simulink model "WaterRunner_open4"  (R2013a)
settings: Solver=ode23s  StartTime=0.0  StopTime=10  RelTol=1e-4
values from neighbouring files (symbols this model uses):
  dTorqueAmp = 1e-2    (= 0.01)    [SimParam_hopper.m]    (also in simParam.m = 0)
  dTorqueFreq = 0.5    [SimParam_hopper.m]    (also in simParam.m = 3.14159265359)
  dWaveAmp = 0    [simParam.m]
  dWaveFreq = (2*pi)/2    (= 3.14159265359)    [simParam.m]
  freq = findSSinput(y,b_water,k_water,A,Fratio,mass*g/4,w0)    [SimParam_hopper.m]    (also in findParams.m = freqs(k); simParam.m; sweepDFomega.m = FREQ(k))
  omega_0 = freq*ones(8,1)    [SimParam_hopper.m]    (also in findParams.m = freq*ones(4,1); simParam.m = freq*ones(4,1); sweepDFomega.m = freq*ones(4,1))
  tail_density = CF_density    (= 1790)    [simParam.m]
  tail_length = 0.1    [simParam.m]
  w1 = freq/(2*df)    [findParams.m]    (also in sweepDFomega.m)
  w2 = freq/(2*(1-df))    [findParams.m]    (also in sweepDFomega.m)
undefined symbols (not defined in the file or in its folder): X, Y, Z
undefined symbols (not defined in the file): cw_FL_HL, cw_FR_FL, cw_FR_HR, cw_HR_HL, FL_HL_lag, FR_FL_lag, FR_HR_lag, HR_HL_lag, phi0, tail_pad_radius, theta0, water_level, y0
libraries: nesl_utility x35, sm_lib x34, WaterRunner_lib_2 x11, simulink x2
(part 2 of 4)

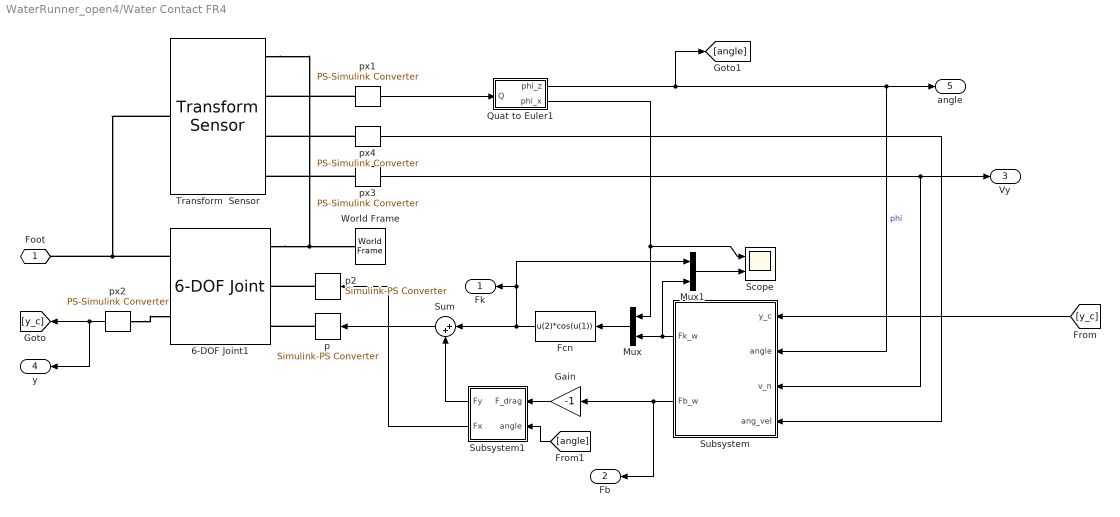
== system WaterRunner_open4/Water Contact FR4 ==
  6-DOF Joint1 : sm_lib/Joints/6-DOF Joint  SenseConstraintForceX=off  SenseConstraintForceY=off  SenseConstraintForceZ=off  SenseConstraintTorqueX=off  SenseConstraintTorqueY=off  SenseConstraintTorqueZ=off  ConstraintWrenchDir=FollowerOnBase  ConstraintWrenchFrame=BaseFrame  PxEquilibriumPosition=0  PxEquilibriumPositionUnits=m  PxSpringStiffness=0  PxSpringStiffnessUnits=N/m  PxDampingCoefficient=0  PxDampingCoefficientUnits=N/(m/s)  PxActuationMode=TorqueForceActuation  PxSensePosition=off  PxSenseVelocity=off  PxSenseAcceleration=off  PxSenseTorqueForce=off  PxPositionTargetValue=0  PxPositionTargetValueUnits=m  PxPositionTargetSpecify=off  PxPositionTargetPriority=High  PxVelocityTargetValue=0  PxVelocityTargetValueUnits=m/s  PxVelocityTargetSpecify=off  PxVelocityTargetPriority=High  PyEquilibriumPosition=0  PyEquilibriumPositionUnits=m  PySpringStiffness=0  PySpringStiffnessUnits=N/m  PyDampingCoefficient=0  PyDampingCoefficientUnits=N/(m/s)  PyActuationMode=TorqueForceActuation  PySensePosition=on  PySenseVelocity=off  PySenseAcceleration=off  PySenseTorqueForce=off  PyPositionTargetValue=0  PyPositionTargetValueUnits=m  PyPositionTargetSpecify=off  PyPositionTargetPriority=High  PyVelocityTargetValue=0  PyVelocityTargetValueUnits=m/s  PyVelocityTargetSpecify=off  PyVelocityTargetPriority=High  PzEquilibriumPosition=0  PzEquilibriumPositionUnits=m  PzSpringStiffness=0  PzSpringStiffnessUnits=N/m  PzDampingCoefficient=0  PzDampingCoefficientUnits=N/(m/s)  PzActuationMode=NoActuation  PzSensePosition=off  PzSenseVelocity=off  PzSenseAcceleration=off  PzSenseTorqueForce=off  PzPositionTargetValue=0  PzPositionTargetValueUnits=m  PzPositionTargetSpecify=off  PzPositionTargetPriority=High  PzVelocityTargetValue=0  PzVelocityTargetValueUnits=m/s  PzVelocityTargetSpecify=off  PzVelocityTargetPriority=High  SphDefPosRotationMethod=None  SphDefPosRotationAngleUnits=deg  SphDefPosRotationStandardAxis=+Z  SphDefPosRotationAngle=0  SphDefPosRotationArbitraryAxis=[0 0 1]  SphDefPosFollAlignAxisA=+X  SphDefPosBaseAlignAxisA=+Y  SphDefPosFollAlignAxisB=+Y  SphDefPosBaseAlignAxisB=+Z  SphEqPosRotationMethod=None  SphEqPosRotationAngleUnits=deg  SphEqPosRotationStandardAxis=+Z  SphEqPosRotationAngle=0  SphEqPosRotationArbitraryAxis=[0 0 1]  SphEqPosFollAlignAxisA=+X  SphEqPosBaseAlignAxisA=+Y  SphEqPosFollAlignAxisB=+Y  SphEqPosBaseAlignAxisB=+Z  SphSpringStiffness=0  SphSpringStiffnessUnits=N*m/deg  SphDampingCoefficient=0  SphDampingCoefficientUnits=N*m/(deg/s)  SphActuateTorqueX=off  SphActuateTorqueY=off  SphActuateTorqueZ=off  SphActuateTorque=off  SphActuationMode=NoActuation  SphActuationFrame=BaseFrame  SphSensePosition=off  SphSenseVelocityX=off  SphSenseVelocityY=off  SphSenseVelocityZ=off  SphSenseVelocity=off  SphSenseAccelerationX=off  SphSenseAccelerationY=off  SphSenseAccelerationZ=off  SphSenseAcceleration=off  SphSenseTorqueX=off  SphSenseTorqueY=off  SphSenseTorqueZ=off  SphSenseTorqueForce=off  SphSensingFrame=BaseFrame  SphPositionTargetRotationMethod=None  SphPositionTargetRotationAngleUnits=deg  SphPositionTargetRotationStandardAxis=+Z  SphPositionTargetRotationAngle=0  SphPositionTargetRotationArbitraryAxis=[0 0 1]  SphPositionTargetFollAlignAxisA=+X  SphPositionTargetBaseAlignAxisA=+Y  SphPositionTargetFollAlignAxisB=+Y  SphPositionTargetBaseAlignAxisB=+Z  SphPositionTargetSpecify=off  SphPositionTargetPriority=High  SphVelocityTargetValue=[0 0 0]  SphVelocityTargetValueUnits=deg/s  SphVelocityTargetSpecify=off  SphVelocityTargetPriority=High  SphVelocityTargetInFollowerFrame=on  BlockFunction=simmechanics.library.joints.sixdof_joint
  Fcn : Fcn  Expr=u(2)*cos(u(1))
  Gain : Gain  Gain=-1
  Mux : Mux  Inputs=2
  Mux1 : Mux  Inputs=2
  Quat to Euler1 : Subsystem
  Scope : Scope  NumInputPorts=2
      settings: YMin=-0.19~0  YMax=0.04~0.7  SaveName=ScopeData3
  Subsystem : Subsystem
  Subsystem1 : Subsystem
  Sum : Sum  Inputs=|++
  Transform  Sensor : sm_lib/Frames and  Transforms/Transform  Sensor  MeasurementFrame=NonRotatingBase  SenseAngle=off  SenseAxis=off  SenseAngle1=off  SenseAngle2=off  SenseAngle3=off  SenseQ=on  SenseR=off  SenseOmegaX=off  SenseOmegaY=off  SenseOmegaZ=on  SenseOmega1=off  SenseOmega2=off  SenseOmega3=off  SenseQDot=off  SenseRDot=off  SenseAlphaX=off  SenseAlphaY=off  SenseAlphaZ=off  SenseAlpha1=off  SenseAlpha2=off  SenseAlpha3=off  SenseQDDot=off  SenseRDDot=off  SenseX=off  SenseY=off  SenseZ=off  SenseRad=off  SenseAzim=off  SenseDist=off  SenseInc=off  SenseXDot=off  SenseYDot=on  SenseZDot=off  SenseRadDot=off  SenseAzimDot=off  SenseDistDot=off  SenseIncDot=off  SenseXDDot=off  SenseYDDot=off  SenseZDDot=off  SenseRadDDot=off  SenseAzimDDot=off  SenseDistDDot=off  SenseIncDDot=off  BlockFunction=simmechanics.library.frames_transforms.transform_sensor
  World Frame : sm_lib/Frames and  Transforms/World Frame  BlockFunction=simmechanics.library.frames_transforms.world_frame
  p : nesl_utility/Simulink-PS Converter  PhysicalDomain=network_engine_domain  SubClassName=ps_input  LeftPortType=input  RightPortType=output  PseudoPeriodic=off  Frequencies=[]  NoiseDistribution=none  NoiseParameters=[]  Unit=1  AffineConversion=off  InputFiltering=off  SimscapeFilterOrder=1  InputFilterTimeConstant=.001  UdotUserProvided=[]
  p2 : nesl_utility/Simulink-PS Converter  PhysicalDomain=network_engine_domain  SubClassName=ps_input  LeftPortType=input  RightPortType=output  PseudoPeriodic=off  Frequencies=[]  NoiseDistribution=none  NoiseParameters=[]  Unit=1  AffineConversion=off  InputFiltering=off  SimscapeFilterOrder=1  InputFilterTimeConstant=.001  UdotUserProvided=[]
  px{1..4} (4 alike) : nesl_utility/PS-Simulink Converter  PhysicalDomain=network_engine_domain  SubClassName=ps_output  LeftPortType=input  RightPortType=output  PseudoPeriodic=off  Frequencies=[]  Unit=1  AffineConversion=off
  Foot : PMIOPort  Port=1  Side=Left
  Fk : Outport
  Fb : Outport  Port=2
  Vy : Outport  Port=3
  y : Outport  Port=4
  angle : Outport  Port=5
  wires:
  Subsystem/2(Fb_w) -> Gain/1, Fb/1
  px3/1 -> Vy/1, Subsystem/3(v_n)
  Quat to Euler1/1(phi_z) -> [angle], Subsystem/2(angle), angle/1  "phi"
  px1/1 -> Quat to Euler1/1(Q)
  px4/1 -> Subsystem/4(ang_vel)
  px2/1 -> [y_c], y/1
  [angle] -> Subsystem1/2(angle)
  Sum/1 -> p/1
  Subsystem1/1(Fy) -> Sum/2
  Gain/1 -> Subsystem1/1(F_drag)
  Subsystem1/2(Fx) -> p2/1
  Subsystem/1(Fk_w) -> Mux1/2, Mux/2
  Mux/1 -> Fcn/1
  Fcn/1 -> Mux1/1, Fk/1, Sum/1
  Quat to Euler1/2(phi_x) -> Mux/1, Scope/1
  Mux1/1 -> Scope/2
  [y_c] -> Subsystem/1(y_c)
  connections:
  Transform  Sensor/RConn1 -- World Frame/RConn1 -- 6-DOF Joint1/LConn1
  Transform  Sensor/LConn1 -- Foot/RConn1 -- 6-DOF Joint1/RConn1
  px2/LConn1 -- 6-DOF Joint1/RConn2
  p/RConn1 -- 6-DOF Joint1/LConn3
  px1/LConn1 -- Transform  Sensor/RConn2
  p2/RConn1 -- 6-DOF Joint1/LConn2
  px3/LConn1 -- Transform  Sensor/RConn4
  px4/LConn1 -- Transform  Sensor/RConn3

== system WaterRunner_open4/observer ==
  Gain : Gain  Gain=-1
  Integrator : Integrator
  Integrator1 : Integrator
  Mux : Mux  Inputs=2
  Mux5 : Mux  Inputs=2
  PS-Simulink Converter : nesl_utility/PS-Simulink Converter  PhysicalDomain=network_engine_domain  SubClassName=ps_output  LeftPortType=input  RightPortType=output  PseudoPeriodic=off  Frequencies=[]  Unit=1  AffineConversion=off
  PS-Simulink Converter1 : nesl_utility/PS-Simulink Converter  PhysicalDomain=network_engine_domain  SubClassName=ps_output  LeftPortType=input  RightPortType=output  PseudoPeriodic=off  Frequencies=[]  Unit=1  AffineConversion=off
  PS-Simulink Converter2 : nesl_utility/PS-Simulink Converter  PhysicalDomain=network_engine_domain  SubClassName=ps_output  LeftPortType=input  RightPortType=output  PseudoPeriodic=off  Frequencies=[]  Unit=1  AffineConversion=off
  Transform  Sensor : sm_lib/Frames and  Transforms/Transform  Sensor  MeasurementFrame=World  SenseAngle=off  SenseAxis=off  SenseAngle1=off  SenseAngle2=off  SenseAngle3=off  SenseQ=off  SenseR=off  SenseOmegaX=on  SenseOmegaY=off  SenseOmegaZ=on  SenseOmega1=off  SenseOmega2=off  SenseOmega3=off  SenseQDot=off  SenseRDot=off  SenseAlphaX=off  SenseAlphaY=off  SenseAlphaZ=off  SenseAlpha1=off  SenseAlpha2=off  SenseAlpha3=off  SenseQDDot=off  SenseRDDot=off  SenseX=off  SenseY=on  SenseZ=off  SenseRad=off  SenseAzim=off  SenseDist=off  SenseInc=off  SenseXDot=off  SenseYDot=off  SenseZDot=off  SenseRadDot=off  SenseAzimDot=off  SenseDistDot=off  SenseIncDot=off  SenseXDDot=off  SenseYDDot=off  SenseZDDot=off  SenseRadDDot=off  SenseAzimDDot=off  SenseDistDDot=off  SenseIncDDot=off  BlockFunction=simmechanics.library.frames_transforms.transform_sensor
  averaging1 : Subsystem  mask{T_win=2*pi/freq, x_init=y0}
      mask prompts: T_win "window (s)"; x_init "Initial condition"
  averaging5 : Subsystem  mask{T_win=2*pi/freq, x_init=[theta0 phi0]}
      mask prompts: T_win "window (s)"; x_init "Initial condition"
  Base : PMIOPort  Port=1  Side=Left
  Follower : PMIOPort  Port=2  Side=Left
  output : Outport
  wires:
  Mux5/1 -> output/1
  Mux/1 -> averaging5/1(in)
  PS-Simulink Converter/1 -> Integrator/1
  Integrator1/1 -> Mux/2
  Integrator/1 -> Gain/1
  PS-Simulink Converter1/1 -> Integrator1/1
  PS-Simulink Converter2/1 -> averaging1/1(in)
  averaging1/1(out) -> Mux5/1
  averaging5/1(out) -> Mux5/2
  Gain/1 -> Mux/1
  connections:
  Transform  Sensor/LConn1 -- Base/RConn1
  PS-Simulink Converter/LConn1 -- Transform  Sensor/RConn2
  Follower/RConn1 -- Transform  Sensor/RConn1
  PS-Simulink Converter1/LConn1 -- Transform  Sensor/RConn3
  PS-Simulink Converter2/LConn1 -- Transform  Sensor/RConn4

== system WaterRunner_open4/CPG_Network/FL_HL lag ==
  In1 : Inport
  In2 : Inport  Port=2
  Constant : Constant  Value=d_phase
  Gain : Gain  Gain=-1
  Sum : Sum  Inputs=--+
  sin : Fcn  Expr=coupling_weight*sin(u(1))
  Out1 : Outport
  Out2 : Outport  Port=2
  wires:
  Sum/1 -> sin/1
  sin/1 -> Gain/1, Out1/1
  Constant/1 -> Sum/2
  In1/1 -> Sum/1
  In2/1 -> Sum/3
  Gain/1 -> Out2/1

== system WaterRunner_open4/CPG_Network/FR_FL lag ==
  In1 : Inport
  In2 : Inport  Port=2
  Constant : Constant  Value=d_phase
  Gain : Gain  Gain=-1
  Sum : Sum  Inputs=--+
  sin : Fcn  Expr=coupling_weight*sin(u(1))
  Out1 : Outport
  Out2 : Outport  Port=2
  wires:
  Sum/1 -> sin/1
  sin/1 -> Gain/1, Out1/1
  Constant/1 -> Sum/2
  In1/1 -> Sum/1
  In2/1 -> Sum/3
  Gain/1 -> Out2/1

== system WaterRunner_open4/CPG_Network/FR_HR lag ==
  In1 : Inport
  In2 : Inport  Port=2
  Constant : Constant  Value=d_phase
  Gain : Gain  Gain=-1
  Sum : Sum  Inputs=--+
  sin : Fcn  Expr=coupling_weight*sin(u(1))
  Out1 : Outport
  Out2 : Outport  Port=2
  wires:
  Gain/1 -> Out2/1
  In2/1 -> Sum/3
  In1/1 -> Sum/1
  Constant/1 -> Sum/2
  sin/1 -> Out1/1, Gain/1
  Sum/1 -> sin/1

== system WaterRunner_open4/CPG_Network/Front_Left ==
  force : Inport
  Constant3 : Constant  Value=freq
  Integrator3 : Integrator  InitialCondition=init_phi + 0.001*rand
  Mod 2pi : Fcn  Expr=atan2(sin(u(1)-pi),cos(u(1)-pi))+pi
  Sum2 : Sum  Inputs=|++
  vel : Outport
  phase : Outport  Port=2
  wires:
  force/1 -> Sum2/2
  Sum2/1 -> vel/1, Integrator3/1
  Constant3/1 -> Sum2/1
  Integrator3/1 -> Mod 2pi/1
  Mod 2pi/1 -> phase/1

== system WaterRunner_open4/CPG_Network/Front_Right ==
  force : Inport
  Constant3 : Constant  Value=freq
  Integrator3 : Integrator  InitialCondition=init_phi + 0.001*rand
  Mod 2pi : Fcn  Expr=atan2(sin(u(1)-pi),cos(u(1)-pi))+pi
  Sum2 : Sum  Inputs=|++
  vel : Outport
  phase : Outport  Port=2
  wires:
  Mod 2pi/1 -> phase/1
  Integrator3/1 -> Mod 2pi/1
  Constant3/1 -> Sum2/1
  Sum2/1 -> Integrator3/1, vel/1
  force/1 -> Sum2/2

== system WaterRunner_open4/CPG_Network/HR_HL lag ==
  In1 : Inport
  In2 : Inport  Port=2
  Constant : Constant  Value=d_phase
  Gain : Gain  Gain=-1
  Sum : Sum  Inputs=--+
  sin : Fcn  Expr=coupling_weight*sin(u(1))
  Out1 : Outport
  Out2 : Outport  Port=2
  wires:
  Gain/1 -> Out2/1
  In2/1 -> Sum/3
  In1/1 -> Sum/1
  Constant/1 -> Sum/2
  sin/1 -> Out1/1, Gain/1
  Sum/1 -> sin/1

== system WaterRunner_open4/CPG_Network/Hind_Left ==
  force : Inport
  Constant3 : Constant  Value=freq
  Integrator3 : Integrator  InitialCondition=init_phi + 0.001*rand
  Mod 2pi : Fcn  Expr=atan2(sin(u(1)-pi),cos(u(1)-pi))+pi
  Sum2 : Sum  Inputs=|++
  vel : Outport
  phase : Outport  Port=2
  wires:
  force/1 -> Sum2/2
  Sum2/1 -> vel/1, Integrator3/1
  Constant3/1 -> Sum2/1
  Integrator3/1 -> Mod 2pi/1
  Mod 2pi/1 -> phase/1

== system WaterRunner_open4/CPG_Network/Hind_Right ==
  force : Inport
  Constant3 : Constant  Value=freq
  Integrator3 : Integrator  InitialCondition=init_phi + 0.001*rand
  Mod 2pi : Fcn  Expr=atan2(sin(u(1)-pi),cos(u(1)-pi))+pi
  Sum2 : Sum  Inputs=|++
  vel : Outport
  phase : Outport  Port=2
  wires:
  force/1 -> Sum2/2
  Sum2/1 -> vel/1, Integrator3/1
  Constant3/1 -> Sum2/1
  Integrator3/1 -> Mod 2pi/1
  Mod 2pi/1 -> phase/1

== system WaterRunner_open4/CPG_Network/split FL ==
  w_pos : Inport
  phase : Inport  Port=2
  w_neg : Inport  Port=3
  Product : Product  RndMeth=Zero
  Product1 : Product  RndMeth=Zero
  Sum2 : Sum  Inputs=|++
  enable : Subsystem
  Force : Outport
  wires:
  Product/1 -> Sum2/1
  w_pos/1 -> Product/1
  w_neg/1 -> Product1/1
  Product1/1 -> Sum2/2
  enable/1(pos) -> Product/2
  enable/2(neg) -> Product1/2
  Sum2/1 -> Force/1
  phase/1 -> enable/1(in)

== system WaterRunner_open4/CPG_Network/split FL1 ==
  w_pos : Inport
  phase : Inport  Port=2
  w_neg : Inport  Port=3
  Product : Product  RndMeth=Zero
  Product1 : Product  RndMeth=Zero
  Sum2 : Sum  Inputs=|++
  enable : Subsystem
  Force : Outport
  wires:
  Product/1 -> Sum2/1
  w_pos/1 -> Product/1
  w_neg/1 -> Product1/1
  Product1/1 -> Sum2/2
  enable/1(pos) -> Product/2
  enable/2(neg) -> Product1/2
  Sum2/1 -> Force/1
  phase/1 -> enable/1(in)

== system WaterRunner_open4/CPG_Network/split FL2 ==
  w_pos : Inport
  phase : Inport  Port=2
  w_neg : Inport  Port=3
  Product : Product  RndMeth=Zero
  Product1 : Product  RndMeth=Zero
  Sum2 : Sum  Inputs=|++
  enable : Subsystem
  Force : Outport
  wires:
  phase/1 -> enable/1(in)
  Sum2/1 -> Force/1
  enable/2(neg) -> Product1/2
  enable/1(pos) -> Product/2
  Product1/1 -> Sum2/2
  w_neg/1 -> Product1/1
  w_pos/1 -> Product/1
  Product/1 -> Sum2/1

== system WaterRunner_open4/CPG_Network/split FL3 ==
  w_pos : Inport
  phase : Inport  Port=2
  w_neg : Inport  Port=3
  Product : Product  RndMeth=Zero
  Product1 : Product  RndMeth=Zero
  Sum2 : Sum  Inputs=|++
  enable : Subsystem
  Force : Outport
  wires:
  Product/1 -> Sum2/1
  w_pos/1 -> Product/1
  w_neg/1 -> Product1/1
  Product1/1 -> Sum2/2
  enable/1(pos) -> Product/2
  enable/2(neg) -> Product1/2
  Sum2/1 -> Force/1
  phase/1 -> enable/1(in)

== system WaterRunner_open4/Tail/Water Contact HR1 ==
  6-DOF Joint2 : sm_lib/Joints/6-DOF Joint  SenseConstraintForceX=off  SenseConstraintForceY=off  SenseConstraintForceZ=off  SenseConstraintTorqueX=off  SenseConstraintTorqueY=off  SenseConstraintTorqueZ=off  ConstraintWrenchDir=FollowerOnBase  ConstraintWrenchFrame=BaseFrame  PxEquilibriumPosition=0  PxEquilibriumPositionUnits=m  PxSpringStiffness=0  PxSpringStiffnessUnits=N/m  PxDampingCoefficient=0  PxDampingCoefficientUnits=N/(m/s)  PxActuationMode=TorqueForceActuation  PxSensePosition=off  PxSenseVelocity=off  PxSenseAcceleration=off  PxSenseTorqueForce=off  PxPositionTargetValue=0  PxPositionTargetValueUnits=m  PxPositionTargetSpecify=off  PxPositionTargetPriority=High  PxVelocityTargetValue=0  PxVelocityTargetValueUnits=m/s  PxVelocityTargetSpecify=off  PxVelocityTargetPriority=High  PyEquilibriumPosition=0  PyEquilibriumPositionUnits=m  PySpringStiffness=0  PySpringStiffnessUnits=N/m  PyDampingCoefficient=0  PyDampingCoefficientUnits=N/(m/s)  PyActuationMode=TorqueForceActuation  PySensePosition=on  PySenseVelocity=off  PySenseAcceleration=off  PySenseTorqueForce=off  PyPositionTargetValue=0  PyPositionTargetValueUnits=m  PyPositionTargetSpecify=off  PyPositionTargetPriority=High  PyVelocityTargetValue=0  PyVelocityTargetValueUnits=m/s  PyVelocityTargetSpecify=off  PyVelocityTargetPriority=High  PzEquilibriumPosition=0  PzEquilibriumPositionUnits=m  PzSpringStiffness=0  PzSpringStiffnessUnits=N/m  PzDampingCoefficient=0  PzDampingCoefficientUnits=N/(m/s)  PzActuationMode=NoActuation  PzSensePosition=off  PzSenseVelocity=off  PzSenseAcceleration=off  PzSenseTorqueForce=off  PzPositionTargetValue=0  PzPositionTargetValueUnits=m  PzPositionTargetSpecify=off  PzPositionTargetPriority=High  PzVelocityTargetValue=0  PzVelocityTargetValueUnits=m/s  PzVelocityTargetSpecify=off  PzVelocityTargetPriority=High  SphDefPosRotationMethod=None  SphDefPosRotationAngleUnits=deg  SphDefPosRotationStandardAxis=+Z  SphDefPosRotationAngle=0  SphDefPosRotationArbitraryAxis=[0 0 1]  SphDefPosFollAlignAxisA=+X  SphDefPosBaseAlignAxisA=+Y  SphDefPosFollAlignAxisB=+Y  SphDefPosBaseAlignAxisB=+Z  SphEqPosRotationMethod=None  SphEqPosRotationAngleUnits=deg  SphEqPosRotationStandardAxis=+Z  SphEqPosRotationAngle=0  SphEqPosRotationArbitraryAxis=[0 0 1]  SphEqPosFollAlignAxisA=+X  SphEqPosBaseAlignAxisA=+Y  SphEqPosFollAlignAxisB=+Y  SphEqPosBaseAlignAxisB=+Z  SphSpringStiffness=0  SphSpringStiffnessUnits=N*m/deg  SphDampingCoefficient=0  SphDampingCoefficientUnits=N*m/(deg/s)  SphActuateTorqueX=off  SphActuateTorqueY=off  SphActuateTorqueZ=off  SphActuateTorque=off  SphActuationMode=NoActuation  SphActuationFrame=BaseFrame  SphSensePosition=off  SphSenseVelocityX=off  SphSenseVelocityY=off  SphSenseVelocityZ=off  SphSenseVelocity=off  SphSenseAccelerationX=off  SphSenseAccelerationY=off  SphSenseAccelerationZ=off  SphSenseAcceleration=off  SphSenseTorqueX=off  SphSenseTorqueY=off  SphSenseTorqueZ=off  SphSenseTorqueForce=off  SphSensingFrame=BaseFrame  SphPositionTargetRotationMethod=None  SphPositionTargetRotationAngleUnits=deg  SphPositionTargetRotationStandardAxis=+Z  SphPositionTargetRotationAngle=0  SphPositionTargetRotationArbitraryAxis=[0 0 1]  SphPositionTargetFollAlignAxisA=+X  SphPositionTargetBaseAlignAxisA=+Y  SphPositionTargetFollAlignAxisB=+Y  SphPositionTargetBaseAlignAxisB=+Z  SphPositionTargetSpecify=off  SphPositionTargetPriority=High  SphVelocityTargetValue=[0 0 0]  SphVelocityTargetValueUnits=deg/s  SphVelocityTargetSpecify=off  SphVelocityTargetPriority=High  SphVelocityTargetInFollowerFrame=on  BlockFunction=simmechanics.library.joints.sixdof_joint
  Gain : Gain  Gain=-1
  Gain1 : Gain  Gain=-1
  Quat to Euler1 : WaterRunner_lib_2/Water Contact FR/Quat to Euler1
  Subsystem1 : WaterRunner_lib_2/Water Contact FR/Subsystem1
  Transform  Sensor : sm_lib/Frames and  Transforms/Transform  Sensor  MeasurementFrame=NonRotatingBase  SenseAngle=off  SenseAxis=off  SenseAngle1=off  SenseAngle2=off  SenseAngle3=off  SenseQ=on  SenseR=off  SenseOmegaX=off  SenseOmegaY=off  SenseOmegaZ=on  SenseOmega1=off  SenseOmega2=off  SenseOmega3=off  SenseQDot=off  SenseRDot=off  SenseAlphaX=off  SenseAlphaY=off  SenseAlphaZ=off  SenseAlpha1=off  SenseAlpha2=off  SenseAlpha3=off  SenseQDDot=off  SenseRDDot=off  SenseX=off  SenseY=off  SenseZ=off  SenseRad=off  SenseAzim=off  SenseDist=off  SenseInc=off  SenseXDot=off  SenseYDot=on  SenseZDot=off  SenseRadDot=off  SenseAzimDot=off  SenseDistDot=off  SenseIncDot=off  SenseXDDot=off  SenseYDDot=off  SenseZDDot=off  SenseRadDDot=off  SenseAzimDDot=off  SenseDistDDot=off  SenseIncDDot=off  BlockFunction=simmechanics.library.frames_transforms.transform_sensor
  World Frame1 : sm_lib/Frames and  Transforms/World Frame  BlockFunction=simmechanics.library.frames_transforms.world_frame
  p : nesl_utility/Simulink-PS Converter  PhysicalDomain=network_engine_domain  SubClassName=ps_input  LeftPortType=input  RightPortType=output  PseudoPeriodic=off  Frequencies=[]  NoiseDistribution=none  NoiseParameters=[]  Unit=1  AffineConversion=off  InputFiltering=off  SimscapeFilterOrder=1  InputFilterTimeConstant=.001  UdotUserProvided=[]
  p2 : nesl_utility/Simulink-PS Converter  PhysicalDomain=network_engine_domain  SubClassName=ps_input  LeftPortType=input  RightPortType=output  PseudoPeriodic=off  Frequencies=[]  NoiseDistribution=none  NoiseParameters=[]  Unit=1  AffineConversion=off  InputFiltering=off  SimscapeFilterOrder=1  InputFilterTimeConstant=.001  UdotUserProvided=[]
  px{1..4} (4 alike) : nesl_utility/PS-Simulink Converter  PhysicalDomain=network_engine_domain  SubClassName=ps_output  LeftPortType=input  RightPortType=output  PseudoPeriodic=off  Frequencies=[]  Unit=1  AffineConversion=off
  water_model : Subsystem  mask{Cd=0.703, density=1000, y_w=water_level, R=tail_pad_radius, g=-9.81}
      mask prompts: Cd "Drag Coefficient"; y_w "Water level"; R "Foot Radius"; g "Gravity constant (use negative)"
  Foot : PMIOPort  Port=1  Side=Left
  Fb : Outport
  wires:
  water_model/1(Fb_w) -> Fb/1, Gain/1
  px3/1 -> water_model/3(v_n)
  Quat to Euler1/1 -> [angle], water_model/2(angle)  "phi"
  px1/1 -> Quat to Euler1/1
  px4/1 -> water_model/4(ang_vel)
  px2/1 -> [y_c]
  [y_c] -> water_model/1(y_c)
  [angle] -> Subsystem1/2
  Subsystem1/2 -> Gain1/1
  Subsystem1/1 -> p/1
  Gain/1 -> Subsystem1/1
  Gain1/1 -> p2/1
  connections:
  World Frame1/RConn1 -- Transform  Sensor/RConn1 -- 6-DOF Joint2/LConn1
  Transform  Sensor/LConn1 -- Foot/RConn1 -- 6-DOF Joint2/RConn1
  Transform  Sensor/RConn4 -- px3/LConn1
  px4/LConn1 -- Transform  Sensor/RConn3
  p2/RConn1 -- 6-DOF Joint2/LConn2
  p/RConn1 -- 6-DOF Joint2/LConn3
  px2/LConn1 -- 6-DOF Joint2/RConn2
  px1/LConn1 -- Transform  Sensor/RConn2

== system WaterRunner_open4/Water Contact FR1/Quat to Euler1 ==
  Q : Inport
  f1 : Fcn  Expr=atan2( 2*(u(1)*u(2) + u(3)*u(4)) , 1-2*(u(2)^2+u(3)^2) )
  f3 : Fcn  Expr=atan2( 2*(u(1)*u(4) + u(2)*u(3)) , 1-2*(u(3)^2+u(4)^2) )
  phi_z : Outport
  phi_x : Outport  Port=2
  wires:
  Q/1 -> f1/1, f3/1
  f3/1 -> phi_z/1
  f1/1 -> phi_x/1

== system WaterRunner_open4/Water Contact FR1/Subsystem ==
  y_c : Inport
  angle : Inport  Port=2
  v_n : Inport  Port=3
  ang_vel : Inport  Port=4
  Switch : Switch
  Switch1 : Switch
  water_model : Subsystem  mask{Cd=0.703, density=1000, y_w=water_level, R=0.02, g=-9.81}
      mask prompts: Cd "Drag Coefficient"; y_w "Water level"; R "Foot Radius"; g "Gravity constant (use negative)"
  water_model1 : Subsystem  mask{Cd=0.703, density=1000, y_w=water_level, R=0.005, g=-9.81}
      mask prompts: Cd "Drag Coefficient"; y_w "Water level"; R "Foot Radius"; g "Gravity constant (use negative)"
  Fk_w : Outport
  Fb_w : Outport  Port=2
  wires:
  angle/1 -> water_model1/2(angle), water_model/2(angle)
  ang_vel/1 -> water_model1/4(ang_vel), water_model/4(ang_vel)
  y_c/1 -> water_model1/1(y_c), water_model/1(y_c)
  v_n/1 -> water_model1/3(v_n), Switch/2, Switch1/2, water_model/3(v_n)
  water_model/1(Fk_w) -> Switch/1
  water_model/2(Fb_w) -> Switch1/1
  Switch/1 -> Fk_w/1
  water_model1/1(Fk_w) -> Switch/3
  water_model1/2(Fb_w) -> Switch1/3
  Switch1/1 -> Fb_w/1

== system WaterRunner_open4/Water Contact FR1/Subsystem1 ==
  F_drag : Inport
  angle : Inport  Port=2
  Mux : Mux  Inputs=2
  fcosq : Fcn  Expr=u(1)*cos(u(2))
  fsinq : Fcn  Expr=u(1)*sin(u(2))
  Fy : Outport
  Fx : Outport  Port=2
  wires:
  angle/1 -> Mux/2
  fcosq/1 -> Fy/1
  F_drag/1 -> Mux/1
  Mux/1 -> fcosq/1, fsinq/1
  fsinq/1 -> Fx/1

== system WaterRunner_open4/Water Contact FR2/Quat to Euler1 ==
  Q : Inport
  f1 : Fcn  Expr=atan2( 2*(u(1)*u(2) + u(3)*u(4)) , 1-2*(u(2)^2+u(3)^2) )
  f3 : Fcn  Expr=atan2( 2*(u(1)*u(4) + u(2)*u(3)) , 1-2*(u(3)^2+u(4)^2) )
  phi_z : Outport
  phi_x : Outport  Port=2
  wires:
  Q/1 -> f1/1, f3/1
  f3/1 -> phi_z/1
  f1/1 -> phi_x/1

== system WaterRunner_open4/Water Contact FR2/Subsystem ==
  y_c : Inport
  angle : Inport  Port=2
  v_n : Inport  Port=3
  ang_vel : Inport  Port=4
  Switch : Switch
  Switch1 : Switch
  water_model : Subsystem  mask{Cd=0.703, density=1000, y_w=water_level, R=0.02, g=-9.81}
      mask prompts: Cd "Drag Coefficient"; y_w "Water level"; R "Foot Radius"; g "Gravity constant (use negative)"
  water_model1 : Subsystem  mask{Cd=0.703, density=1000, y_w=water_level, R=0.005, g=-9.81}
      mask prompts: Cd "Drag Coefficient"; y_w "Water level"; R "Foot Radius"; g "Gravity constant (use negative)"
  Fk_w : Outport
  Fb_w : Outport  Port=2
  wires:
  angle/1 -> water_model1/2(angle), water_model/2(angle)
  ang_vel/1 -> water_model1/4(ang_vel), water_model/4(ang_vel)
  y_c/1 -> water_model1/1(y_c), water_model/1(y_c)
  v_n/1 -> water_model1/3(v_n), Switch/2, Switch1/2, water_model/3(v_n)
  water_model/1(Fk_w) -> Switch/1
  water_model/2(Fb_w) -> Switch1/1
  Switch/1 -> Fk_w/1
  water_model1/1(Fk_w) -> Switch/3
  water_model1/2(Fb_w) -> Switch1/3
  Switch1/1 -> Fb_w/1

== system WaterRunner_open4/Water Contact FR2/Subsystem1 ==
  F_drag : Inport
  angle : Inport  Port=2
  Mux : Mux  Inputs=2
  fcosq : Fcn  Expr=u(1)*cos(u(2))
  fsinq : Fcn  Expr=u(1)*sin(u(2))
  Fy : Outport
  Fx : Outport  Port=2
  wires:
  angle/1 -> Mux/2
  fcosq/1 -> Fy/1
  F_drag/1 -> Mux/1
  Mux/1 -> fcosq/1, fsinq/1
  fsinq/1 -> Fx/1

== system WaterRunner_open4/Water Contact FR3/Quat to Euler1 ==
  Q : Inport
  f1 : Fcn  Expr=atan2( 2*(u(1)*u(2) + u(3)*u(4)) , 1-2*(u(2)^2+u(3)^2) )
  f3 : Fcn  Expr=atan2( 2*(u(1)*u(4) + u(2)*u(3)) , 1-2*(u(3)^2+u(4)^2) )
  phi_z : Outport
  phi_x : Outport  Port=2
  wires:
  Q/1 -> f1/1, f3/1
  f3/1 -> phi_z/1
  f1/1 -> phi_x/1

== system WaterRunner_open4/Water Contact FR3/Subsystem ==
  y_c : Inport
  angle : Inport  Port=2
  v_n : Inport  Port=3
  ang_vel : Inport  Port=4
  Switch : Switch
  Switch1 : Switch
  water_model : Subsystem  mask{Cd=0.703, density=1000, y_w=water_level, R=0.02, g=-9.81}
      mask prompts: Cd "Drag Coefficient"; y_w "Water level"; R "Foot Radius"; g "Gravity constant (use negative)"
  water_model1 : Subsystem  mask{Cd=0.703, density=1000, y_w=water_level, R=0.005, g=-9.81}
      mask prompts: Cd "Drag Coefficient"; y_w "Water level"; R "Foot Radius"; g "Gravity constant (use negative)"
  Fk_w : Outport
  Fb_w : Outport  Port=2
  wires:
  angle/1 -> water_model1/2(angle), water_model/2(angle)
  ang_vel/1 -> water_model1/4(ang_vel), water_model/4(ang_vel)
  y_c/1 -> water_model1/1(y_c), water_model/1(y_c)
  v_n/1 -> water_model1/3(v_n), Switch/2, Switch1/2, water_model/3(v_n)
  water_model/1(Fk_w) -> Switch/1
  water_model/2(Fb_w) -> Switch1/1
  Switch/1 -> Fk_w/1
  water_model1/1(Fk_w) -> Switch/3
  water_model1/2(Fb_w) -> Switch1/3
  Switch1/1 -> Fb_w/1

== system WaterRunner_open4/Water Contact FR3/Subsystem1 ==
  F_drag : Inport
  angle : Inport  Port=2
  Mux : Mux  Inputs=2
  fcosq : Fcn  Expr=u(1)*cos(u(2))
  fsinq : Fcn  Expr=u(1)*sin(u(2))
  Fy : Outport
  Fx : Outport  Port=2
  wires:
  angle/1 -> Mux/2
  fcosq/1 -> Fy/1
  F_drag/1 -> Mux/1
  Mux/1 -> fcosq/1, fsinq/1
  fsinq/1 -> Fx/1

== system WaterRunner_open4/Water Contact FR4/Quat to Euler1 ==
  Q : Inport
  f1 : Fcn  Expr=atan2( 2*(u(1)*u(2) + u(3)*u(4)) , 1-2*(u(2)^2+u(3)^2) )
  f3 : Fcn  Expr=atan2( 2*(u(1)*u(4) + u(2)*u(3)) , 1-2*(u(3)^2+u(4)^2) )
  phi_z : Outport
  phi_x : Outport  Port=2
  wires:
  Q/1 -> f1/1, f3/1
  f3/1 -> phi_z/1
  f1/1 -> phi_x/1

== system WaterRunner_open4/Water Contact FR4/Subsystem ==
  y_c : Inport
  angle : Inport  Port=2
  v_n : Inport  Port=3
  ang_vel : Inport  Port=4
  Switch : Switch
  Switch1 : Switch
  water_model : Subsystem  mask{Cd=0.703, density=1000, y_w=water_level, R=0.02, g=-9.81}
      mask prompts: Cd "Drag Coefficient"; y_w "Water level"; R "Foot Radius"; g "Gravity constant (use negative)"
  water_model1 : Subsystem  mask{Cd=0.703, density=1000, y_w=water_level, R=0.005, g=-9.81}
      mask prompts: Cd "Drag Coefficient"; y_w "Water level"; R "Foot Radius"; g "Gravity constant (use negative)"
  Fk_w : Outport
  Fb_w : Outport  Port=2
  wires:
  angle/1 -> water_model1/2(angle), water_model/2(angle)
  ang_vel/1 -> water_model1/4(ang_vel), water_model/4(ang_vel)
  y_c/1 -> water_model1/1(y_c), water_model/1(y_c)
  v_n/1 -> water_model1/3(v_n), Switch/2, Switch1/2, water_model/3(v_n)
  water_model/1(Fk_w) -> Switch/1
  water_model/2(Fb_w) -> Switch1/1
  Switch/1 -> Fk_w/1
  water_model1/1(Fk_w) -> Switch/3
  water_model1/2(Fb_w) -> Switch1/3
  Switch1/1 -> Fb_w/1

== system WaterRunner_open4/Water Contact FR4/Subsystem1 ==
  F_drag : Inport
  angle : Inport  Port=2
  Mux : Mux  Inputs=2
  fcosq : Fcn  Expr=u(1)*cos(u(2))
  fsinq : Fcn  Expr=u(1)*sin(u(2))
  Fy : Outport
  Fx : Outport  Port=2
  wires:
  angle/1 -> Mux/2
  fcosq/1 -> Fy/1
  F_drag/1 -> Mux/1
  Mux/1 -> fcosq/1, fsinq/1
  fsinq/1 -> Fx/1

== system WaterRunner_open4/observer/averaging1 ==
  in : Inport
  Constant1 : Constant  Value=x_init
  Gain : Gain  Gain=1/T_win
  Integrator1 : Integrator
  Sum : Sum  Inputs=+-|
  Sum1 : Sum  Inputs=-+|
  Sum3 : Sum  Inputs=++|
  Transport Delay : TransportDelay  DelayTime=T_win
  out : Outport
  wires:
  in/1 -> Sum1/2
  Gain/1 -> Sum3/2
  Constant1/1 -> Sum3/1, Sum1/1
  Sum1/1 -> Integrator1/1
  Transport Delay/1 -> Sum/2
  Integrator1/1 -> Sum/1, Transport Delay/1
  Sum3/1 -> out/1
  Sum/1 -> Gain/1

== system WaterRunner_open4/observer/averaging5 ==
  in : Inport
  Constant1 : Constant  Value=x_init
  Gain : Gain  Gain=1/T_win
  Integrator1 : Integrator
  Sum : Sum  Inputs=+-|
  Sum1 : Sum  Inputs=-+|
  Sum3 : Sum  Inputs=++|
  Transport Delay : TransportDelay  DelayTime=T_win
  out : Outport
  wires:
  in/1 -> Sum1/2
  Gain/1 -> Sum3/2
  Constant1/1 -> Sum3/1, Sum1/1
  Sum1/1 -> Integrator1/1
  Transport Delay/1 -> Sum/2
  Integrator1/1 -> Sum/1, Transport Delay/1
  Sum3/1 -> out/1
  Sum/1 -> Gain/1

== system WaterRunner_open4/CPG_Network/split FL/enable ==
  in : Inport
  Constant1 : Constant
  Constant2 : Constant
  Fcn : Fcn  Expr=cos(u(1))
  Gain : Gain  Gain=.5
  Gain1 : Gain  Gain=.5
  Sign : Signum
  Sum1 : Sum  Inputs=|++
  Sum2 : Sum  Inputs=|-+
  pos : Outport
  neg : Outport  Port=2
  wires:
  Fcn/1 -> Sign/1
  Constant1/1 -> Sum1/2
  Sign/1 -> Sum2/1, Sum1/1
  Gain/1 -> pos/1
  in/1 -> Fcn/1
  Sum1/1 -> Gain/1
  Constant2/1 -> Sum2/2
  Gain1/1 -> neg/1
  Sum2/1 -> Gain1/1

== system WaterRunner_open4/CPG_Network/split FL1/enable ==
  in : Inport
  Constant1 : Constant
  Constant2 : Constant
  Fcn : Fcn  Expr=cos(u(1))
  Gain : Gain  Gain=.5
  Gain1 : Gain  Gain=.5
  Sign : Signum
  Sum1 : Sum  Inputs=|++
  Sum2 : Sum  Inputs=|-+
  pos : Outport
  neg : Outport  Port=2
  wires:
  Fcn/1 -> Sign/1
  Constant1/1 -> Sum1/2
  Sign/1 -> Sum2/1, Sum1/1
  Gain/1 -> pos/1
  in/1 -> Fcn/1
  Sum1/1 -> Gain/1
  Constant2/1 -> Sum2/2
  Gain1/1 -> neg/1
  Sum2/1 -> Gain1/1

== system WaterRunner_open4/CPG_Network/split FL2/enable ==
  in : Inport
  Constant1 : Constant
  Constant2 : Constant
  Fcn : Fcn  Expr=cos(u(1))
  Gain : Gain  Gain=.5
  Gain1 : Gain  Gain=.5
  Sign : Signum
  Sum1 : Sum  Inputs=|++
  Sum2 : Sum  Inputs=|-+
  pos : Outport
  neg : Outport  Port=2
  wires:
  Sum2/1 -> Gain1/1
  Gain1/1 -> neg/1
  Constant2/1 -> Sum2/2
  Sum1/1 -> Gain/1
  in/1 -> Fcn/1
  Gain/1 -> pos/1
  Sign/1 -> Sum1/1, Sum2/1
  Constant1/1 -> Sum1/2
  Fcn/1 -> Sign/1

== system WaterRunner_open4/CPG_Network/split FL3/enable ==
  in : Inport
  Constant1 : Constant
  Constant2 : Constant
  Fcn : Fcn  Expr=cos(u(1))
  Gain : Gain  Gain=.5
  Gain1 : Gain  Gain=.5
  Sign : Signum
  Sum1 : Sum  Inputs=|++
  Sum2 : Sum  Inputs=|-+
  pos : Outport
  neg : Outport  Port=2
  wires:
  Fcn/1 -> Sign/1
  Constant1/1 -> Sum1/2
  Sign/1 -> Sum2/1, Sum1/1
  Gain/1 -> pos/1
  in/1 -> Fcn/1
  Sum1/1 -> Gain/1
  Constant2/1 -> Sum2/2
  Gain1/1 -> neg/1
  Sum2/1 -> Gain1/1

== system WaterRunner_open4/Tail/Water Contact HR1/water_model ==
  y_c : Inport
  angle : Inport  Port=2
  v_n : Inport  Port=3
  ang_vel : Inport  Port=4
  Gain1 : Gain  Gain=Cd*density
  Gain3 : Gain  Gain=-1
  Product1 : Product  RndMeth=Zero
  Product2 : Product  RndMeth=Zero
  Subsystem : Subsystem
  Subsystem1 : Subsystem
  Subsystem2 : Subsystem
  Subsystem3 : Subsystem
  Sum : Sum  Inputs=|++
  Sum2 : Sum  Inputs=-+|
  damper_force1 : Subsystem
  damper_force2 : Subsystem
  Fb_w : Outport
  wires:
  Gain1/1 -> Gain3/1
  Sum/1 -> Gain1/1
  Product2/1 -> Sum/2
  ang_vel/1 -> damper_force1/2(a), damper_force2/2(a), Subsystem3/2(dtheta), Subsystem2/1(dtheta)
  v_n/1 -> damper_force1/3(b), damper_force2/3(b), Subsystem3/1(vel), Subsystem2/2(v)
  angle/1 -> Subsystem/2(angle)
  y_c/1 -> Subsystem/1(y_c)
  Product1/1 -> Sum/1
  damper_force2/1(Int_b) -> Product1/1
  damper_force1/1(Int_b) -> Product2/1
  Subsystem2/1(S+) -> Sum2/1, Product1/2
  Subsystem2/2(S-) -> Sum2/2
  Sum2/1 -> Product2/2
  Subsystem3/1(mid_b) -> Subsystem2/3(r0), Subsystem1/2(r0)
  Gain3/1 -> Fb_w/1
  Subsystem/1(up_b) -> damper_force2/1(up_b), Subsystem1/1(r)
  Subsystem1/1(r00) -> damper_force1/1(up_b)

== system WaterRunner_open4/Water Contact FR1/Subsystem/water_model ==
  y_c : Inport
  angle : Inport  Port=2
  v_n : Inport  Port=3
  ang_vel : Inport  Port=4
  Gain : Gain
  Gain1 : Gain  Gain=Cd*density
  Gain2 : Gain  Gain=Cd*density
  Gain3 : Gain  Gain=-1
  Product1 : Product  RndMeth=Zero
  Product2 : Product  RndMeth=Zero
  Subsystem : Subsystem
  Subsystem1 : Subsystem
  Subsystem2 : Subsystem
  Subsystem3 : Subsystem
  Subsystem4 : Subsystem
  Sum : Sum  Inputs=|++
  Sum2 : Sum  Inputs=-+|
  damper_force1 : Subsystem
  damper_force2 : Subsystem
  spring_force : Subsystem
  Fk_w : Outport
  Fb_w : Outport  Port=2
  wires:
  Subsystem4/1(r00) -> damper_force1/1(up_b)
  Subsystem3/1(mid_b) -> Subsystem4/2(r0), Subsystem2/3(r0)
  Gain1/1 -> Gain3/1
  Sum/1 -> Gain1/1
  Product2/1 -> Sum/2
  Subsystem1/2(b) -> spring_force/3(b)
  spring_force/1(Int_k) -> Gain2/1
  Gain2/1 -> Gain/1
  ang_vel/1 -> damper_force1/2(a), damper_force2/2(a), Subsystem3/2(dtheta), Subsystem2/1(dtheta)
  v_n/1 -> damper_force1/3(b), damper_force2/3(b), Subsystem3/1(vel), Subsystem2/2(v)
  Subsystem1/1(a) -> spring_force/2(a)
  angle/1 -> Subsystem/2(angle), Subsystem1/2(angle)
  y_c/1 -> Subsystem/1(y_c), Subsystem1/1(y_c)
  Subsystem/1(up_b) -> damper_force2/1(up_b), Subsystem4/1(r), spring_force/1(up_b)
  Product1/1 -> Sum/1
  damper_force2/1(Int_b) -> Product1/1
  damper_force1/1(Int_b) -> Product2/1
  Subsystem2/1(S+) -> Sum2/1, Product1/2
  Subsystem2/2(S-) -> Sum2/2
  Sum2/1 -> Product2/2
  Gain/1 -> Fk_w/1
  Gain3/1 -> Fb_w/1

== system WaterRunner_open4/Water Contact FR1/Subsystem/water_model1 ==
  y_c : Inport
  angle : Inport  Port=2
  v_n : Inport  Port=3
  ang_vel : Inport  Port=4
  Gain : Gain
  Gain1 : Gain  Gain=Cd*density
  Gain2 : Gain  Gain=Cd*density
  Gain3 : Gain  Gain=-1
  Product1 : Product  RndMeth=Zero
  Product2 : Product  RndMeth=Zero
  Subsystem : Subsystem
  Subsystem1 : Subsystem
  Subsystem2 : Subsystem
  Subsystem3 : Subsystem
  Subsystem4 : Subsystem
  Sum : Sum  Inputs=|++
  Sum2 : Sum  Inputs=-+|
  damper_force1 : Subsystem
  damper_force2 : Subsystem
  spring_force : Subsystem
  Fk_w : Outport
  Fb_w : Outport  Port=2
  wires:
  Subsystem4/1(r00) -> damper_force1/1(up_b), Subsystem2/3(r0)
  Subsystem3/1(mid_b) -> Subsystem4/2(r0)
  Gain1/1 -> Gain3/1
  Sum/1 -> Gain1/1
  Product2/1 -> Sum/2
  Subsystem1/2(b) -> spring_force/3(b)
  spring_force/1(Int_k) -> Gain2/1
  Gain2/1 -> Gain/1
  ang_vel/1 -> damper_force1/2(a), damper_force2/2(a), Subsystem3/2(dtheta), Subsystem2/1(dtheta)
  v_n/1 -> damper_force1/3(b), damper_force2/3(b), Subsystem3/1(vel), Subsystem2/2(v)
  Subsystem1/1(a) -> spring_force/2(a)
  angle/1 -> Subsystem/2(angle), Subsystem1/2(angle)
  y_c/1 -> Subsystem/1(y_c), Subsystem1/1(y_c)
  Subsystem/1(up_b) -> damper_force2/1(up_b), Subsystem4/1(r), spring_force/1(up_b)
  Product1/1 -> Sum/1
  damper_force2/1(Int_b) -> Product1/1
  damper_force1/1(Int_b) -> Product2/1
  Subsystem2/1(S+) -> Sum2/1, Product1/2
  Subsystem2/2(S-) -> Sum2/2
  Sum2/1 -> Product2/2
  Gain/1 -> Fk_w/1
  Gain3/1 -> Fb_w/1

== system WaterRunner_open4/Water Contact FR2/Subsystem/water_model ==
  y_c : Inport
  angle : Inport  Port=2
  v_n : Inport  Port=3
  ang_vel : Inport  Port=4
  Gain : Gain
  Gain1 : Gain  Gain=Cd*density
  Gain2 : Gain  Gain=Cd*density
  Gain3 : Gain  Gain=-1
  Product1 : Product  RndMeth=Zero
  Product2 : Product  RndMeth=Zero
  Subsystem : Subsystem
  Subsystem1 : Subsystem
  Subsystem2 : Subsystem
  Subsystem3 : Subsystem
  Subsystem4 : Subsystem
  Sum : Sum  Inputs=|++
  Sum2 : Sum  Inputs=-+|
  damper_force1 : Subsystem
  damper_force2 : Subsystem
  spring_force : Subsystem
  Fk_w : Outport
  Fb_w : Outport  Port=2
  wires:
  Subsystem4/1(r00) -> damper_force1/1(up_b)
  Subsystem3/1(mid_b) -> Subsystem4/2(r0), Subsystem2/3(r0)
  Gain1/1 -> Gain3/1
  Sum/1 -> Gain1/1
  Product2/1 -> Sum/2
  Subsystem1/2(b) -> spring_force/3(b)
  spring_force/1(Int_k) -> Gain2/1
  Gain2/1 -> Gain/1
  ang_vel/1 -> damper_force1/2(a), damper_force2/2(a), Subsystem3/2(dtheta), Subsystem2/1(dtheta)
  v_n/1 -> damper_force1/3(b), damper_force2/3(b), Subsystem3/1(vel), Subsystem2/2(v)
  Subsystem1/1(a) -> spring_force/2(a)
  angle/1 -> Subsystem/2(angle), Subsystem1/2(angle)
  y_c/1 -> Subsystem/1(y_c), Subsystem1/1(y_c)
  Subsystem/1(up_b) -> damper_force2/1(up_b), Subsystem4/1(r), spring_force/1(up_b)
  Product1/1 -> Sum/1
  damper_force2/1(Int_b) -> Product1/1
  damper_force1/1(Int_b) -> Product2/1
  Subsystem2/1(S+) -> Sum2/1, Product1/2
  Subsystem2/2(S-) -> Sum2/2
  Sum2/1 -> Product2/2
  Gain/1 -> Fk_w/1
  Gain3/1 -> Fb_w/1

== system WaterRunner_open4/Water Contact FR2/Subsystem/water_model1 ==
  y_c : Inport
  angle : Inport  Port=2
  v_n : Inport  Port=3
  ang_vel : Inport  Port=4
  Gain : Gain
  Gain1 : Gain  Gain=Cd*density
  Gain2 : Gain  Gain=Cd*density
  Gain3 : Gain  Gain=-1
  Product1 : Product  RndMeth=Zero
  Product2 : Product  RndMeth=Zero
  Subsystem : Subsystem
  Subsystem1 : Subsystem
  Subsystem2 : Subsystem
  Subsystem3 : Subsystem
  Subsystem4 : Subsystem
  Sum : Sum  Inputs=|++
  Sum2 : Sum  Inputs=-+|
  damper_force1 : Subsystem
  damper_force2 : Subsystem
  spring_force : Subsystem
  Fk_w : Outport
  Fb_w : Outport  Port=2
  wires:
  Subsystem4/1(r00) -> damper_force1/1(up_b), Subsystem2/3(r0)
  Subsystem3/1(mid_b) -> Subsystem4/2(r0)
  Gain1/1 -> Gain3/1
  Sum/1 -> Gain1/1
  Product2/1 -> Sum/2
  Subsystem1/2(b) -> spring_force/3(b)
  spring_force/1(Int_k) -> Gain2/1
  Gain2/1 -> Gain/1
  ang_vel/1 -> damper_force1/2(a), damper_force2/2(a), Subsystem3/2(dtheta), Subsystem2/1(dtheta)
  v_n/1 -> damper_force1/3(b), damper_force2/3(b), Subsystem3/1(vel), Subsystem2/2(v)
  Subsystem1/1(a) -> spring_force/2(a)
  angle/1 -> Subsystem/2(angle), Subsystem1/2(angle)
  y_c/1 -> Subsystem/1(y_c), Subsystem1/1(y_c)
  Subsystem/1(up_b) -> damper_force2/1(up_b), Subsystem4/1(r), spring_force/1(up_b)
  Product1/1 -> Sum/1
  damper_force2/1(Int_b) -> Product1/1
  damper_force1/1(Int_b) -> Product2/1
  Subsystem2/1(S+) -> Sum2/1, Product1/2
  Subsystem2/2(S-) -> Sum2/2
  Sum2/1 -> Product2/2
  Gain/1 -> Fk_w/1
  Gain3/1 -> Fb_w/1

== system WaterRunner_open4/Water Contact FR3/Subsystem/water_model ==
  y_c : Inport
  angle : Inport  Port=2
  v_n : Inport  Port=3
  ang_vel : Inport  Port=4
  Gain : Gain
  Gain1 : Gain  Gain=Cd*density
  Gain2 : Gain  Gain=Cd*density
  Gain3 : Gain  Gain=-1
  Product1 : Product  RndMeth=Zero
  Product2 : Product  RndMeth=Zero
  Subsystem : Subsystem
  Subsystem1 : Subsystem
  Subsystem2 : Subsystem
  Subsystem3 : Subsystem
  Subsystem4 : Subsystem
  Sum : Sum  Inputs=|++
  Sum2 : Sum  Inputs=-+|
  damper_force1 : Subsystem
  damper_force2 : Subsystem
  spring_force : Subsystem
  Fk_w : Outport
  Fb_w : Outport  Port=2
  wires:
  Subsystem4/1(r00) -> damper_force1/1(up_b)
  Subsystem3/1(mid_b) -> Subsystem4/2(r0), Subsystem2/3(r0)
  Gain1/1 -> Gain3/1
  Sum/1 -> Gain1/1
  Product2/1 -> Sum/2
  Subsystem1/2(b) -> spring_force/3(b)
  spring_force/1(Int_k) -> Gain2/1
  Gain2/1 -> Gain/1
  ang_vel/1 -> damper_force1/2(a), damper_force2/2(a), Subsystem3/2(dtheta), Subsystem2/1(dtheta)
  v_n/1 -> damper_force1/3(b), damper_force2/3(b), Subsystem3/1(vel), Subsystem2/2(v)
  Subsystem1/1(a) -> spring_force/2(a)
  angle/1 -> Subsystem/2(angle), Subsystem1/2(angle)
  y_c/1 -> Subsystem/1(y_c), Subsystem1/1(y_c)
  Subsystem/1(up_b) -> damper_force2/1(up_b), Subsystem4/1(r), spring_force/1(up_b)
  Product1/1 -> Sum/1
  damper_force2/1(Int_b) -> Product1/1
  damper_force1/1(Int_b) -> Product2/1
  Subsystem2/1(S+) -> Sum2/1, Product1/2
  Subsystem2/2(S-) -> Sum2/2
  Sum2/1 -> Product2/2
  Gain/1 -> Fk_w/1
  Gain3/1 -> Fb_w/1

== system WaterRunner_open4/Water Contact FR3/Subsystem/water_model1 ==
  y_c : Inport
  angle : Inport  Port=2
  v_n : Inport  Port=3
  ang_vel : Inport  Port=4
  Gain : Gain
  Gain1 : Gain  Gain=Cd*density
  Gain2 : Gain  Gain=Cd*density
  Gain3 : Gain  Gain=-1
  Product1 : Product  RndMeth=Zero
  Product2 : Product  RndMeth=Zero
  Subsystem : Subsystem
  Subsystem1 : Subsystem
  Subsystem2 : Subsystem
  Subsystem3 : Subsystem
  Subsystem4 : Subsystem
  Sum : Sum  Inputs=|++
  Sum2 : Sum  Inputs=-+|
  damper_force1 : Subsystem
  damper_force2 : Subsystem
  spring_force : Subsystem
  Fk_w : Outport
  Fb_w : Outport  Port=2
  wires:
  Subsystem4/1(r00) -> damper_force1/1(up_b), Subsystem2/3(r0)
  Subsystem3/1(mid_b) -> Subsystem4/2(r0)
  Gain1/1 -> Gain3/1
  Sum/1 -> Gain1/1
  Product2/1 -> Sum/2
  Subsystem1/2(b) -> spring_force/3(b)
  spring_force/1(Int_k) -> Gain2/1
  Gain2/1 -> Gain/1
  ang_vel/1 -> damper_force1/2(a), damper_force2/2(a), Subsystem3/2(dtheta), Subsystem2/1(dtheta)
  v_n/1 -> damper_force1/3(b), damper_force2/3(b), Subsystem3/1(vel), Subsystem2/2(v)
  Subsystem1/1(a) -> spring_force/2(a)
  angle/1 -> Subsystem/2(angle), Subsystem1/2(angle)
  y_c/1 -> Subsystem/1(y_c), Subsystem1/1(y_c)
  Subsystem/1(up_b) -> damper_force2/1(up_b), Subsystem4/1(r), spring_force/1(up_b)
  Product1/1 -> Sum/1
  damper_force2/1(Int_b) -> Product1/1
  damper_force1/1(Int_b) -> Product2/1
  Subsystem2/1(S+) -> Sum2/1, Product1/2
  Subsystem2/2(S-) -> Sum2/2
  Sum2/1 -> Product2/2
  Gain/1 -> Fk_w/1
  Gain3/1 -> Fb_w/1

== system WaterRunner_open4/Water Contact FR4/Subsystem/water_model ==
  y_c : Inport
  angle : Inport  Port=2
  v_n : Inport  Port=3
  ang_vel : Inport  Port=4
  Gain : Gain
  Gain1 : Gain  Gain=Cd*density
  Gain2 : Gain  Gain=Cd*density
  Gain3 : Gain  Gain=-1
  Product1 : Product  RndMeth=Zero
  Product2 : Product  RndMeth=Zero
  Subsystem : Subsystem
  Subsystem1 : Subsystem
  Subsystem2 : Subsystem
  Subsystem3 : Subsystem
  Subsystem4 : Subsystem
  Sum : Sum  Inputs=|++
  Sum2 : Sum  Inputs=-+|
  damper_force1 : Subsystem
  damper_force2 : Subsystem
  spring_force : Subsystem
  Fk_w : Outport
  Fb_w : Outport  Port=2
  wires:
  Subsystem4/1(r00) -> damper_force1/1(up_b)
  Subsystem3/1(mid_b) -> Subsystem4/2(r0), Subsystem2/3(r0)
  Gain1/1 -> Gain3/1
  Sum/1 -> Gain1/1
  Product2/1 -> Sum/2
  Subsystem1/2(b) -> spring_force/3(b)
  spring_force/1(Int_k) -> Gain2/1
  Gain2/1 -> Gain/1
  ang_vel/1 -> damper_force1/2(a), damper_force2/2(a), Subsystem3/2(dtheta), Subsystem2/1(dtheta)
  v_n/1 -> damper_force1/3(b), damper_force2/3(b), Subsystem3/1(vel), Subsystem2/2(v)
  Subsystem1/1(a) -> spring_force/2(a)
  angle/1 -> Subsystem/2(angle), Subsystem1/2(angle)
  y_c/1 -> Subsystem/1(y_c), Subsystem1/1(y_c)
  Subsystem/1(up_b) -> damper_force2/1(up_b), Subsystem4/1(r), spring_force/1(up_b)
  Product1/1 -> Sum/1
  damper_force2/1(Int_b) -> Product1/1
  damper_force1/1(Int_b) -> Product2/1
  Subsystem2/1(S+) -> Sum2/1, Product1/2
  Subsystem2/2(S-) -> Sum2/2
  Sum2/1 -> Product2/2
  Gain/1 -> Fk_w/1
  Gain3/1 -> Fb_w/1

== system WaterRunner_open4/Water Contact FR4/Subsystem/water_model1 ==
  y_c : Inport
  angle : Inport  Port=2
  v_n : Inport  Port=3
  ang_vel : Inport  Port=4
  Gain : Gain
  Gain1 : Gain  Gain=Cd*density
  Gain2 : Gain  Gain=Cd*density
  Gain3 : Gain  Gain=-1
  Product1 : Product  RndMeth=Zero
  Product2 : Product  RndMeth=Zero
  Subsystem : Subsystem
  Subsystem1 : Subsystem
  Subsystem2 : Subsystem
  Subsystem3 : Subsystem
  Subsystem4 : Subsystem
  Sum : Sum  Inputs=|++
  Sum2 : Sum  Inputs=-+|
  damper_force1 : Subsystem
  damper_force2 : Subsystem
  spring_force : Subsystem
  Fk_w : Outport
  Fb_w : Outport  Port=2
  wires:
  Subsystem4/1(r00) -> damper_force1/1(up_b), Subsystem2/3(r0)
  Subsystem3/1(mid_b) -> Subsystem4/2(r0)
  Gain1/1 -> Gain3/1
  Sum/1 -> Gain1/1
  Product2/1 -> Sum/2
  Subsystem1/2(b) -> spring_force/3(b)
  spring_force/1(Int_k) -> Gain2/1
  Gain2/1 -> Gain/1
  ang_vel/1 -> damper_force1/2(a), damper_force2/2(a), Subsystem3/2(dtheta), Subsystem2/1(dtheta)
  v_n/1 -> damper_force1/3(b), damper_force2/3(b), Subsystem3/1(vel), Subsystem2/2(v)
  Subsystem1/1(a) -> spring_force/2(a)
  angle/1 -> Subsystem/2(angle), Subsystem1/2(angle)
  y_c/1 -> Subsystem/1(y_c), Subsystem1/1(y_c)
  Subsystem/1(up_b) -> damper_force2/1(up_b), Subsystem4/1(r), spring_force/1(up_b)
  Product1/1 -> Sum/1
  damper_force2/1(Int_b) -> Product1/1
  damper_force1/1(Int_b) -> Product2/1
  Subsystem2/1(S+) -> Sum2/1, Product1/2
  Subsystem2/2(S-) -> Sum2/2
  Sum2/1 -> Product2/2
  Gain/1 -> Fk_w/1
  Gain3/1 -> Fb_w/1

== system WaterRunner_open4/Tail/Water Contact HR1/water_model/Subsystem ==
  note: sign handle the case when angle of tail pass 180 or 0
  y_c : Inport
  angle : Inport  Port=2
  Constant : Constant  Value=y_w
  Fcn : Fcn  Expr=sin(u(1))
  Fcn1 : Fcn  Expr=u(1)/u(2)
  Mux : Mux  Inputs=2
  Product : Product  RndMeth=Zero
  Sign : Signum
  Sum : Sum  Inputs=+-|
  sat : Saturate  UpperLimit=R  LowerLimit=-R
  up_b : Outport
  wires:
  Sum/1 -> Mux/1
  angle/1 -> Fcn/1
  y_c/1 -> Sum/2
  Constant/1 -> Sum/1
  Mux/1 -> Fcn1/1
  Fcn/1 -> Sign/1, Mux/2
  sat/1 -> up_b/1
  Fcn1/1 -> Product/1
  Product/1 -> sat/1
  Sign/1 -> Product/2

== system WaterRunner_open4/Tail/Water Contact HR1/water_model/Subsystem1 ==
  r : Inport
  r0 : Inport  Port=2
  Sum1 : Sum  Inputs=-|+
  Switch : Switch
  r00 : Outport
  wires:
  r/1 -> Sum1/1, Switch/1
  r0/1 -> Sum1/2, Switch/3
  Sum1/1 -> Switch/2
  Switch/1 -> r00/1

== system WaterRunner_open4/Tail/Water Contact HR1/water_model/Subsystem2 ==
  dtheta : Inport
  v : Inport  Port=2
  r0 : Inport  Port=3
  Constant : Constant  Value=2*eps
  Product : Product  RndMeth=Zero
  Product1 : Product  RndMeth=Zero
  Scope3 : Scope  NumInputPorts=4
      settings: TimeRange=0.6  YMin=-0.03~-5~-1~-1  YMax=0.03~4~1~1  SaveName=ScopeData6
  Sign : Signum
  Sign1 : Signum
  Sum2 : Sum  Inputs=|++
  Sum3 : Sum  Inputs=|++
  Sum4 : Sum  Inputs=-+|
  Sum5 : Sum  Inputs=++|
  S+ : Outport
  S- : Outport  Port=2
  wires:
  Product/1 -> Sum2/1
  Product1/1 -> Sum3/1
  Sum5/1 -> Product1/1
  Sign1/1 -> Scope3/4, S-/1
  r0/1 -> Scope3/1, Sum4/2, Sum5/2
  dtheta/1 -> Product/2, Product1/2
  Sign/1 -> Scope3/3, S+/1
  v/1 -> Scope3/2, Sum2/2, Sum3/2
  Sum4/1 -> Product/1
  Constant/1 -> Sum4/1, Sum5/1
  Sum3/1 -> Sign/1
  Sum2/1 -> Sign1/1

== system WaterRunner_open4/Tail/Water Contact HR1/water_model/Subsystem3 ==
  vel : Inport
  dtheta : Inport  Port=2
  C : Constant  Value=0
  Fcn : Fcn  Expr=-u(1)/(u(2))
  Mux : Mux  Inputs=2
  Switch : Switch
  sat1 : Saturate  UpperLimit=R  LowerLimit=-R
  mid_b : Outport
  wires:
  C/1 -> Switch/1
  Switch/1 -> sat1/1
  Fcn/1 -> Switch/3
  sat1/1 -> mid_b/1
  vel/1 -> Mux/1
  dtheta/1 -> Mux/2, Switch/2
  Mux/1 -> Fcn/1
